simulink model "NetworkModelSimpleIntersectionSimpleDroneModel"  (R2018b)
settings: Solver=VariableStepAuto  StartTime=tStart  StopTime=tFinal  FixedStep=0.001  RelTol=1e-3
undefined symbols (not defined in the file or in its folder): bx, by, ConflictDrone1andDrone2, ConflictDrone1andDrone3, ConflictDrone1andDrone4, ConflictDrone2andDrone3, ConflictDrone2andDrone4, ConflictDrone3andDrone4, deltaVx1, deltaVx2, deltaVx3, deltaVx4, deltaVy1, deltaVy2, deltaVy3, deltaVy4, m, VelocityStarX1, VelocityStarX2, VelocityStarX3, VelocityStarX4, VelocityStarY1, VelocityStarY2, VelocityStarY3, VelocityStarY4, vx10, vx20, vx30, vx40, vy10, vy20, vy30, vy40, x10, x20, x30, x40, y10, y20, y30, y40
libraries: simulink x9
settings Model: Creator=CowUser  LastModifiedBy=CowUser

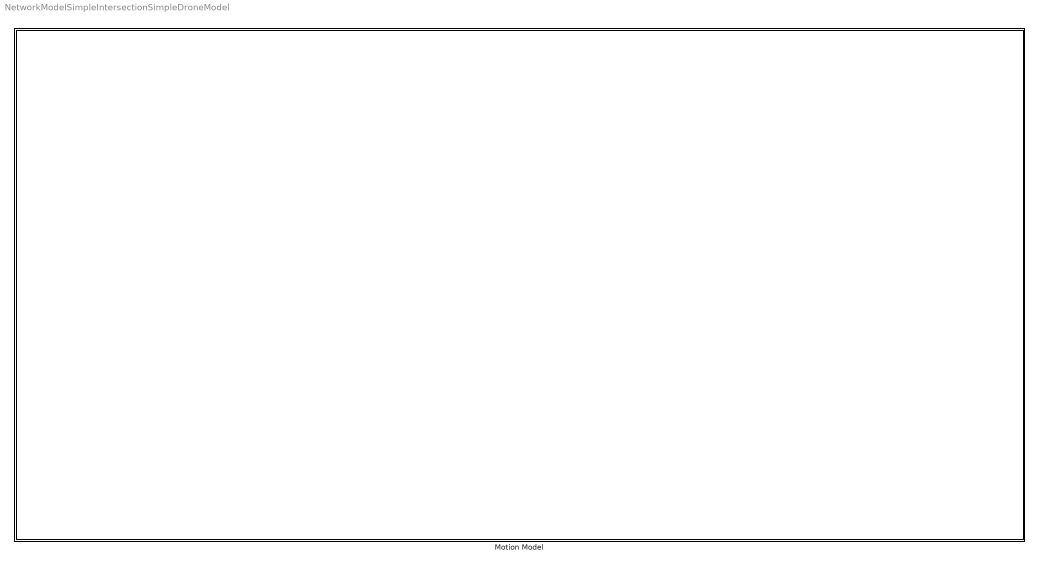
== system NetworkModelSimpleIntersectionSimpleDroneModel ==
  Motion Model : Subsystem

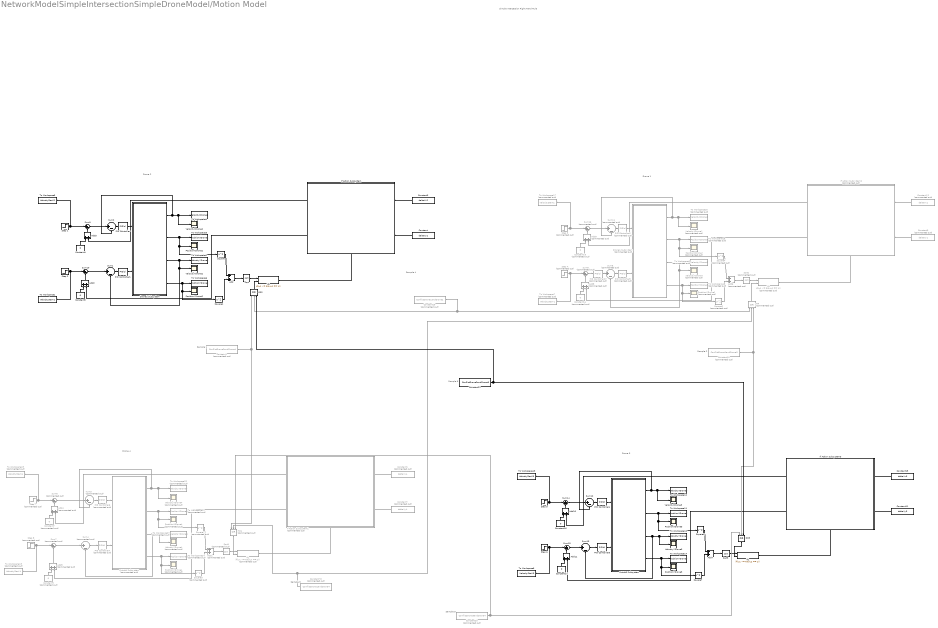
== system NetworkModelSimpleIntersectionSimpleDroneModel/Motion Model ==
  note: Drone 2
  note: Simple Intersection
      |
      | Right Hand Rule
  note: Drone 4
  note: Sample 1
  note: Drone 1
  note: Drone 3
  note: Sample 2
  note: Sample 3
  note: Sample 4
  note: Sample 5
  note: Sample 6
  Add{,2..3,7,10..11} (6 alike) : Sum
  Add{1,4..6,8..9} (6 alike) : Sum  Commented=on
  Constant : Constant  Value=deltaVy2
  Constant1 : Constant  Commented=on  Value=ConflictDrone2andDrone4
  Constant10 : Constant  Commented=on  Value=ConflictDrone1andDrone3
  Constant11 : Constant  Value=deltaVy3
  Constant12 : Constant  Commented=on  Value=deltaVx1
  Constant{7..8,13..14} (4 alike) : Constant  Commented=on  Value=0
  Constant15 : Constant  Value=deltaVx3
  Constant{4..5,16..17} (4 alike) : Constant  Value=0
  Constant18 : Constant  Commented=on  Value=ConflictDrone1andDrone4
  Constant19 : Constant  Commented=on  Value=ConflictDrone1andDrone2
  Constant2 : Constant  Commented=on  Value=deltaVy4
  Constant20 : Constant  Commented=on  Value=ConflictDrone3andDrone4
  Constant21 : Constant  Value=ConflictDrone2andDrone3
  Constant3 : Constant  Value=deltaVx2
  Constant6 : Constant  Commented=on  Value=deltaVx4
  Constant9 : Constant  Commented=on  Value=deltaVy1
  "Drone1 Subsystem " : Subsystem  Commented=on
  "Drone2 Subsystem " : Subsystem
  Drone3 Subsystem : Subsystem
  "Drone4 Subsystem " : Subsystem  Commented=on
  If Action Subsystem : Subsystem  TreatAsAtomicUnit=on
  If Action Subsystem1 : Subsystem  Commented=on  TreatAsAtomicUnit=on
  If Action Subsystem2 : Subsystem  Commented=on  TreatAsAtomicUnit=on
  If Action Subsystem3 : Subsystem  TreatAsAtomicUnit=on
  If1 : If  Commented=on  NumInputs=2  IfExpression=(u1 <= R)&(u2 == 1)  ShowElse=off
  If2 : If  NumInputs=2  IfExpression=(u1 <= R)&(u2 == 1)  ShowElse=off
  If3 : If  NumInputs=2  IfExpression=(u1 <= R)&(u2 == 1)  ShowElse=off
  If4 : If  Commented=on  NumInputs=2  IfExpression=(u1 <= R)&(u2 == 1)  ShowElse=off
  OR : Logic  Commented=on  Operator=OR  Inputs=3  IconShape=distinctive  AllPortsSameDT=off  OutDataTypeStr='double'
  OR1 : Logic  Commented=on  Operator=OR  Inputs=3  IconShape=distinctive  AllPortsSameDT=off  OutDataTypeStr='double'
  OR2 : Logic  Operator=OR  Inputs=3  IconShape=distinctive  AllPortsSameDT=off  OutDataTypeStr='double'
  OR3 : Logic  Operator=OR  Inputs=3  IconShape=distinctive  AllPortsSameDT=off  OutDataTypeStr='double'
  PID Controller{,1,4..5} (4 alike) : simulink/Continuous/PID Controller  Controller=PID  Form=Parallel  TimeDomain=Continuous-time  SampleTime=-1  IntegratorMethod=Forward Euler  FilterMethod=Forward Euler  ControllerParametersSource=internal  P=800  I=40  D=1  UseFilter=on  N=100  TunerSelectOption=Transfer Function Based (PID Tuner App)  InitialConditionSource=internal  InitialConditionForIntegrator=0  InitialConditionForFilter=0  DifferentiatorICPrevScaledInput=0  ExternalReset=none  TrackingMode=off  Kt=1  LimitOutput=off  UpperSaturationLimit=inf  LowerSaturationLimit=-inf  LinearizeAsGain=on  AntiWindupMode=none  Kb=1  POutMin=[]  POutMax=[]  IOutMin=[]  IOutMax=[]  DOutMin=[]  DOutMax=[]  NOutMin=[]  NOutMax=[]  SumOutMin=[]  SumOutMax=[]  SaturationOutMin=[]  SaturationOutMax=[]  PParamMin=[]  PParamMax=[]  IParamMin=[]  IParamMax=[]  DParamMin=[]  DParamMax=[]  NParamMin=[]  NParamMax=[]  KbParamMin=[]  KbParamMax=[]  KtParamMin=[]  KtParamMax=[]  KbOutMin=[]  KbOutMax=[]  KtOutMin=[]  KtOutMax=[]  IntegratorOutMin=[]  IntegratorOutMax=[]  FilterOutMin=[]  FilterOutMax=[]  SumI1OutMin=[]  SumI1OutMax=[]  SumI2OutMin=[]  SumI2OutMax=[]  SumI3OutMin=[]  SumI3OutMax=[]  SumI4OutMin=[]  SumI4OutMax=[]  SumDOutMin=[]  SumDOutMax=[]  DifferentiatorOutMin=[]  DifferentiatorOutMax=[]  FilterDiffOutCoefMin=[]  FilterDiffOutCoefMax=[]  ReciprocalOutMin=[]  ReciprocalOutMax=[]  SumDenOutMin=[]  SumDenOutMax=[]  SumNumOutMin=[]  SumNumOutMax=[]  DivideOutMin=[]  DivideOutMax=[]  IntegratorContinuousStateAttributes=''  IntegratorStateMustResolveToSignalObject=off  IntegratorRTWStateStorageClass=Auto  FilterContinuousStateAttributes=''  FilterStateMustResolveToSignalObject=off  FilterRTWStateStorageClass=Auto  ParallelPVariant=InternalParameters  IdealPVariant=Disabled  IVariant=InternalParameters  DVariant=InternalParameters  IntegratorVariant=Continuous  SatVariant=Disabled  AWVariant=Passthrough  PCopyVariant=Disabled  TRVariant=Disabled  FdbkBlocksVariant=Forward  IdealPFdbkVariant=Disabled  SatFdbkVariant=Disabled  DerivativeFilterVariant=ContFilter  NVariant=InternalParameters  NCopyVariant=Disabled  FilterICVariant=InternalICsFilter  IntegratorICVariant=InternalICs  ExternalResetVariant=Disabled  TRSumVariant=Passthrough  SumFdbkVariant=Disabled  SumVariant=Sum_PID
  PID Controller{2..3,6..7,10} (5 alike) : simulink/Continuous/PID Controller  Commented=on  Controller=PID  Form=Parallel  TimeDomain=Continuous-time  SampleTime=-1  IntegratorMethod=Forward Euler  FilterMethod=Forward Euler  ControllerParametersSource=internal  P=800  I=40  D=1  UseFilter=on  N=100  TunerSelectOption=Transfer Function Based (PID Tuner App)  InitialConditionSource=internal  InitialConditionForIntegrator=0  InitialConditionForFilter=0  DifferentiatorICPrevScaledInput=0  ExternalReset=none  TrackingMode=off  Kt=1  LimitOutput=off  UpperSaturationLimit=inf  LowerSaturationLimit=-inf  LinearizeAsGain=on  AntiWindupMode=none  Kb=1  POutMin=[]  POutMax=[]  IOutMin=[]  IOutMax=[]  DOutMin=[]  DOutMax=[]  NOutMin=[]  NOutMax=[]  SumOutMin=[]  SumOutMax=[]  SaturationOutMin=[]  SaturationOutMax=[]  PParamMin=[]  PParamMax=[]  IParamMin=[]  IParamMax=[]  DParamMin=[]  DParamMax=[]  NParamMin=[]  NParamMax=[]  KbParamMin=[]  KbParamMax=[]  KtParamMin=[]  KtParamMax=[]  KbOutMin=[]  KbOutMax=[]  KtOutMin=[]  KtOutMax=[]  IntegratorOutMin=[]  IntegratorOutMax=[]  FilterOutMin=[]  FilterOutMax=[]  SumI1OutMin=[]  SumI1OutMax=[]  SumI2OutMin=[]  SumI2OutMax=[]  SumI3OutMin=[]  SumI3OutMax=[]  SumI4OutMin=[]  SumI4OutMax=[]  SumDOutMin=[]  SumDOutMax=[]  DifferentiatorOutMin=[]  DifferentiatorOutMax=[]  FilterDiffOutCoefMin=[]  FilterDiffOutCoefMax=[]  ReciprocalOutMin=[]  ReciprocalOutMax=[]  SumDenOutMin=[]  SumDenOutMax=[]  SumNumOutMin=[]  SumNumOutMax=[]  DivideOutMin=[]  DivideOutMax=[]  IntegratorContinuousStateAttributes=''  IntegratorStateMustResolveToSignalObject=off  IntegratorRTWStateStorageClass=Auto  FilterContinuousStateAttributes=''  FilterStateMustResolveToSignalObject=off  FilterRTWStateStorageClass=Auto  ParallelPVariant=InternalParameters  IdealPVariant=Disabled  IVariant=InternalParameters  DVariant=InternalParameters  IntegratorVariant=Continuous  SatVariant=Disabled  AWVariant=Passthrough  PCopyVariant=Disabled  TRVariant=Disabled  FdbkBlocksVariant=Forward  IdealPFdbkVariant=Disabled  SatFdbkVariant=Disabled  DerivativeFilterVariant=ContFilter  NVariant=InternalParameters  NCopyVariant=Disabled  FilterICVariant=InternalICsFilter  IntegratorICVariant=InternalICs  ExternalResetVariant=Disabled  TRSumVariant=Passthrough  SumFdbkVariant=Disabled  SumVariant=Sum_PID
  PositionXDrone1 : Scope  Commented=on
  PositionXDrone2 : Scope
  PositionXDrone3 : Scope
  PositionXDrone4 : Scope  Commented=on
  PositionYDrone1 : Scope  Commented=on
  PositionYDrone2 : Scope
  PositionYDrone3 : Scope
  PositionYDrone4 : Scope  Commented=on
  Sqrt : Sqrt  SaturateOnIntegerOverflow=on
  Sqrt1 : Sqrt  Commented=on  SaturateOnIntegerOverflow=on
  Sqrt2 : Sqrt  Commented=on  SaturateOnIntegerOverflow=on
  Sqrt3 : Sqrt  SaturateOnIntegerOverflow=on
  Square{,1,6..7} (4 alike) : Math  Operator=square  SaturateOnIntegerOverflow=on
  Square{2..5} (4 alike) : Math  Commented=on  Operator=square  SaturateOnIntegerOverflow=on
  Step 1 : Step  Time=0  After=VelocityStarX2  SampleTime=0
  Step 2 : Step  Time=0  After=VelocityStarY2  SampleTime=0
  Step 3 : Step  Commented=on  Time=0  After=VelocityStarX1  SampleTime=0
  Step 4 : Step  Commented=on  Time=0  After=VelocityStarY1  SampleTime=0
  Step 5 : Step  Time=0  After=VelocityStarX3  SampleTime=0
  Step 6 : Step  Time=0  After=VelocityStarY3  SampleTime=0
  Step 7 : Step  Commented=on  Time=0  After=VelocityStarX4  SampleTime=0
  Step 8 : Step  Commented=on  Time=0  After=VelocityStarY4  SampleTime=0
  Sum{1..2,9..10,12..15} (8 alike) : Sum  Inputs=|+-
  Sum{3..8,11,16} (8 alike) : Sum  Commented=on  Inputs=|+-
  To Workspace1 : ToWorkspace  VariableName=VelocityStarY2  SampleTime=-1
  To Workspace10 : ToWorkspace  VariableName=VelocityYDrone3  SampleTime=-1
  To Workspace11 : ToWorkspace  VariableName=PositionXDrone3  SampleTime=-1
  To Workspace12 : ToWorkspace  VariableName=VelocityXDrone3  SampleTime=-1
  To Workspace13 : ToWorkspace  VariableName=VelocityStarX3  SampleTime=-1
  To Workspace14 : ToWorkspace  VariableName=PositionYDrone3  SampleTime=-1
  To Workspace15 : ToWorkspace  Commented=on  VariableName=PositionXDrone1  SampleTime=-1
  To Workspace16 : ToWorkspace  Commented=on  VariableName=VelocityXDrone1  SampleTime=-1
  To Workspace17 : ToWorkspace  Commented=on  VariableName=VelocityStarX1  SampleTime=-1
  To Workspace18 : ToWorkspace  Commented=on  VariableName=PositionYDrone1  SampleTime=-1
  To Workspace19 : ToWorkspace  Commented=on  VariableName=VelocityStarY4  SampleTime=-1
  To Workspace2 : ToWorkspace  VariableName=VelocityYDrone2  SampleTime=-1
  To Workspace20 : ToWorkspace  Commented=on  VariableName=VelocityYDrone4  SampleTime=-1
  To Workspace21 : ToWorkspace  Commented=on  VariableName=PositionXDrone4  SampleTime=-1
  To Workspace22 : ToWorkspace  Commented=on  VariableName=VelocityXDrone4  SampleTime=-1
  To Workspace23 : ToWorkspace  Commented=on  VariableName=VelocityStarX4  SampleTime=-1
  To Workspace24 : ToWorkspace  Commented=on  VariableName=PositionYDrone4  SampleTime=-1
  To Workspace3 : ToWorkspace  VariableName=PositionXDrone2  SampleTime=-1
  To Workspace4 : ToWorkspace  VariableName=VelocityXDrone2  SampleTime=-1
  To Workspace5 : ToWorkspace  VariableName=VelocityStarX2  SampleTime=-1
  To Workspace6 : ToWorkspace  VariableName=PositionYDrone2  SampleTime=-1
  To Workspace7 : ToWorkspace  Commented=on  VariableName=VelocityStarY1  SampleTime=-1
  To Workspace8 : ToWorkspace  VariableName=VelocityStarY3  SampleTime=-1
  To Workspace9 : ToWorkspace  Commented=on  VariableName=VelocityYDrone1  SampleTime=-1
  VelocityXDrone1 : Scope  Commented=on
  VelocityXDrone2 : Scope
  VelocityXDrone3 : Scope
  VelocityXDrone4 : Scope  Commented=on
  VelocityYDrone1 : Scope  Commented=on
  VelocityYDrone2 : Scope
  VelocityYDrone3 : Scope
  VelocityYDrone4 : Scope  Commented=on
  wires:
  "Drone2 Subsystem "/3(VelocityY) -> Sum1/2, VelocityYDrone2/1, To Workspace2/1
  Sum1/1 -> PID Controller1/1
  PID Controller/1 -> "Drone2 Subsystem "/1(InputForceX)
  "Drone2 Subsystem "/4(PositionY) -> Square1/1, PositionYDrone2/1, To Workspace6/1
  "Drone2 Subsystem "/2(PositionX) -> Square/1, PositionXDrone2/1, To Workspace3/1
  PID Controller1/1 -> "Drone2 Subsystem "/2(InputForceY)
  "Drone2 Subsystem "/1(VelocityX) -> VelocityXDrone2/1, To Workspace4/1, Sum2/2
  Step 7/1 -> Sum6/1, To Workspace23/1
  Step 8/1 -> To Workspace19/1, Sum7/1
  Square/1 -> Add/1
  Square1/1 -> Add/2
  Add/1 -> Sqrt/1
  Sqrt/1 -> If3/1
  Square2/1 -> Add1/1
  Add1/1 -> Sqrt1/1
  "Drone4 Subsystem "/2(PositionXTEST) -> Square2/1, PositionXDrone4/1, To Workspace21/1
  Square3/1 -> Add1/2
  "Drone4 Subsystem "/4(PositionYTEST) -> Square3/1, PositionYDrone4/1, To Workspace24/1
  Sqrt1/1 -> If1/1
  Sum2/1 -> PID Controller/1
  Constant/1 -> If Action Subsystem/2(deltaVy2)
  Constant3/1 -> If Action Subsystem/1(deltaVx2)
  Step 1/1 -> Sum9/1, To Workspace5/1
  Sum10/1 -> Sum1/1
  Step 2/1 -> Sum10/1, To Workspace1/1
  If Action Subsystem/1(dVx2) -> Add3/2
  If Action Subsystem/2(dVy2) -> Add2/2
  If3/1 -> If Action Subsystem/Action
  Constant4/1 -> Add3/1
  Constant5/1 -> Add2/1
  Add2/1 -> Sum10/2
  Constant1/1 -> OR1/1, OR2/1
  If1/1 -> If Action Subsystem1/Action
  If Action Subsystem1/1(dVx4) -> Add4/2
  Constant2/1 -> If Action Subsystem1/2(deltaVy4)
  Constant6/1 -> If Action Subsystem1/1(deltaVx4)
  Add4/1 -> Sum6/2
  Constant7/1 -> Add4/1
  Sum3/1 -> PID Controller6/1
  "Drone4 Subsystem "/1(VelocityXTEST) -> Sum3/2, To Workspace22/1, VelocityXDrone4/1
  Constant8/1 -> Add5/1
  If Action Subsystem1/2(dVy4) -> Add5/2
  "Drone4 Subsystem "/3(VelocityYTEST) -> Sum4/2, VelocityYDrone4/1, To Workspace20/1
  Sum4/1 -> PID Controller7/1
  Add3/1 -> Sum9/2
  Sum9/1 -> Sum2/1
  Step 3/1 -> Sum16/1, To Workspace17/1
  Add9/1 -> Sum16/2
  "Drone1 Subsystem "/4(PositionY) -> Square5/1, PositionYDrone1/1, To Workspace18/1
  Drone3 Subsystem/3(VelocityY) -> Sum13/2, VelocityYDrone3/1, To Workspace10/1
  Constant17/1 -> Add11/1
  Add10/1 -> Sum14/2
  Sum15/1 -> Sum13/1
  If Action Subsystem3/2(dVy3) -> Add11/2
  PID Controller2/1 -> "Drone1 Subsystem "/1(InputForceX)
  Add11/1 -> Sum15/2
  Sum11/1 -> PID Controller2/1
  Constant10/1 -> OR3/2, OR/3
  If Action Subsystem2/1(dVx1) -> Add9/2
  Constant11/1 -> If Action Subsystem3/2(deltaVy3)
  Constant13/1 -> Add9/1
  Sqrt3/1 -> If2/1
  Constant16/1 -> Add10/1
  PID Controller3/1 -> "Drone1 Subsystem "/2(InputForceY)
  Add8/1 -> Sum8/2
  Drone3 Subsystem/1(VelocityX) -> Sum12/2, To Workspace12/1, VelocityXDrone3/1
  Constant14/1 -> Add8/1
  If2/1 -> If Action Subsystem3/Action
  If Action Subsystem3/1(dVx3) -> Add10/2
  Drone3 Subsystem/4(PositionY) -> Square7/1, PositionYDrone3/1, To Workspace14/1
  Constant12/1 -> If Action Subsystem2/1(deltaVx1)
  Constant15/1 -> If Action Subsystem3/1(deltaVx3)
  Step 4/1 -> Sum8/1, To Workspace7/1
  "Drone1 Subsystem "/2(PositionX) -> Square4/1, PositionXDrone1/1, To Workspace15/1
  Add7/1 -> Sqrt3/1
  Square6/1 -> Add7/1
  Square5/1 -> Add6/2
  Constant9/1 -> If Action Subsystem2/2(deltaVy1)
  Square7/1 -> Add7/2
  Sum13/1 -> PID Controller5/1
  Drone3 Subsystem/2(PositionX) -> Square6/1, PositionXDrone3/1, To Workspace11/1
  Sum14/1 -> Sum12/1
  Step 5/1 -> Sum14/1, To Workspace13/1
  Sum12/1 -> PID Controller4/1
  Step 6/1 -> To Workspace8/1, Sum15/1
  Sum5/1 -> PID Controller3/1
  Sqrt2/1 -> If4/1
  PID Controller4/1 -> Drone3 Subsystem/1(InputForceX)
  Add6/1 -> Sqrt2/1
  PID Controller5/1 -> Drone3 Subsystem/2(InputForceY)
  "Drone1 Subsystem "/3(VelocityY) -> Sum5/2, VelocityYDrone1/1, To Workspace9/1
  If Action Subsystem2/2(dVy1) -> Add8/2
  Square4/1 -> Add6/1
  If4/1 -> If Action Subsystem2/Action
  "Drone1 Subsystem "/1(VelocityX) -> VelocityXDrone1/1, To Workspace16/1, Sum11/2
  OR/1 -> If4/2
  Constant18/1 -> OR/2, OR1/2
  OR1/1 -> If1/2
  OR2/1 -> If3/2
  Constant19/1 -> OR2/2, OR/1
  Constant20/1 -> OR3/1, OR1/3
  OR3/1 -> If2/2
  Constant21/1 -> OR3/3, OR2/3
  Sum6/1 -> Sum3/1
  PID Controller10/1 -> Sum5/1
  Sum8/1 -> PID Controller10/1
  Sum16/1 -> Sum11/1
  Add5/1 -> Sum7/2
  Sum7/1 -> Sum4/1
  PID Controller6/1 -> "Drone4 Subsystem "/1(InputForceXTEST)
  PID Controller7/1 -> "Drone4 Subsystem "/2(InputForceYTEST)

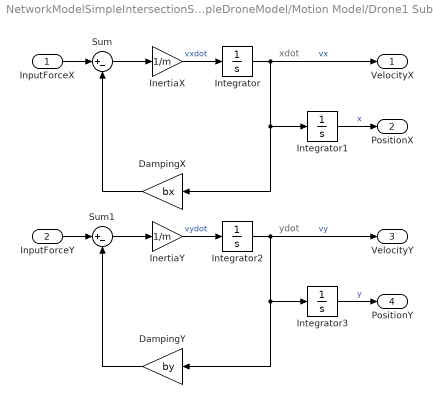
== system NetworkModelSimpleIntersectionSimpleDroneModel/Motion Model/Drone1 Subsystem  ==
  note: xdot
  note: ydot
  InputForceX : Inport
  InputForceY : Inport  Port=2
  "DampingX " : Gain  Gain=bx
  DampingY : Gain  Gain=by
  InertiaX : Gain  Gain=1/m
  InertiaY : Gain  Gain=1/m
  Integrator : Integrator  InitialCondition=vx10
  Integrator1 : Integrator  InitialCondition=x10
  Integrator2 : Integrator  InitialCondition=vy10
  Integrator3 : Integrator  InitialCondition=y10
  Sum : Sum  Inputs=|+-
  Sum1 : Sum  Inputs=|+-
  VelocityX : Outport
  PositionX : Outport  Port=2
  VelocityY : Outport  Port=3
  PositionY : Outport  Port=4
  wires:
  InputForceX/1 -> Sum/1
  InertiaX/1 -> Integrator/1  "vxdot"
  Sum/1 -> InertiaX/1
  Integrator/1 -> VelocityX/1, Integrator1/1, "DampingX "/1  "vx"
  "DampingX "/1 -> Sum/2
  Integrator1/1 -> PositionX/1  "x"
  DampingY/1 -> Sum1/2
  Sum1/1 -> InertiaY/1
  InertiaY/1 -> Integrator2/1  "vydot"
  Integrator3/1 -> PositionY/1  "y"
  InputForceY/1 -> Sum1/1
  Integrator2/1 -> VelocityY/1, Integrator3/1, DampingY/1  "vy"

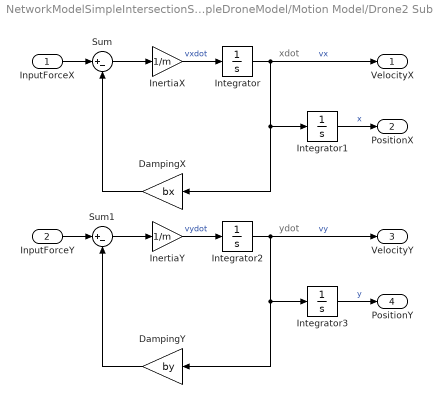
== system NetworkModelSimpleIntersectionSimpleDroneModel/Motion Model/Drone2 Subsystem  ==
  note: xdot
  note: ydot
  InputForceX : Inport
  InputForceY : Inport  Port=2
  "DampingX " : Gain  Gain=bx
  DampingY : Gain  Gain=by
  InertiaX : Gain  Gain=1/m
  InertiaY : Gain  Gain=1/m
  Integrator : Integrator  InitialCondition=vx20
  Integrator1 : Integrator  InitialCondition=x20
  Integrator2 : Integrator  InitialCondition=vy20
  Integrator3 : Integrator  InitialCondition=y20
  Sum : Sum  Inputs=|+-
  Sum1 : Sum  Inputs=|+-
  VelocityX : Outport
  PositionX : Outport  Port=2
  VelocityY : Outport  Port=3
  PositionY : Outport  Port=4
  wires:
  InputForceX/1 -> Sum/1
  InertiaX/1 -> Integrator/1  "vxdot"
  Sum/1 -> InertiaX/1
  Integrator/1 -> VelocityX/1, Integrator1/1, "DampingX "/1  "vx"
  "DampingX "/1 -> Sum/2
  Integrator1/1 -> PositionX/1  "x"
  DampingY/1 -> Sum1/2
  Sum1/1 -> InertiaY/1
  InertiaY/1 -> Integrator2/1  "vydot"
  Integrator3/1 -> PositionY/1  "y"
  InputForceY/1 -> Sum1/1
  Integrator2/1 -> VelocityY/1, Integrator3/1, DampingY/1  "vy"

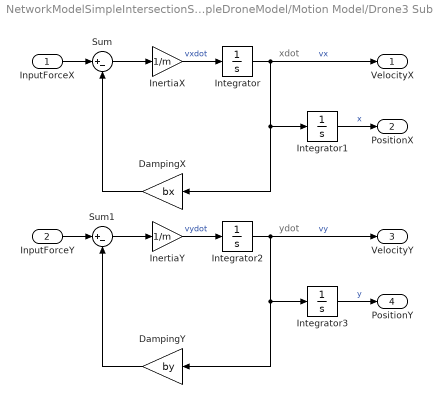
== system NetworkModelSimpleIntersectionSimpleDroneModel/Motion Model/Drone3 Subsystem ==
  note: xdot
  note: ydot
  InputForceX : Inport
  InputForceY : Inport  Port=2
  "DampingX " : Gain  Gain=bx
  DampingY : Gain  Gain=by
  InertiaX : Gain  Gain=1/m
  InertiaY : Gain  Gain=1/m
  Integrator : Integrator  InitialCondition=vx30
  Integrator1 : Integrator  InitialCondition=x30
  Integrator2 : Integrator  InitialCondition=vy30
  Integrator3 : Integrator  InitialCondition=y30
  Sum : Sum  Inputs=|+-
  Sum1 : Sum  Inputs=|+-
  VelocityX : Outport
  PositionX : Outport  Port=2
  VelocityY : Outport  Port=3
  PositionY : Outport  Port=4
  wires:
  InputForceX/1 -> Sum/1
  InertiaX/1 -> Integrator/1  "vxdot"
  Sum/1 -> InertiaX/1
  Integrator/1 -> VelocityX/1, Integrator1/1, "DampingX "/1  "vx"
  "DampingX "/1 -> Sum/2
  Integrator1/1 -> PositionX/1  "x"
  DampingY/1 -> Sum1/2
  Sum1/1 -> InertiaY/1
  InertiaY/1 -> Integrator2/1  "vydot"
  Integrator3/1 -> PositionY/1  "y"
  InputForceY/1 -> Sum1/1
  Integrator2/1 -> VelocityY/1, Integrator3/1, DampingY/1  "vy"

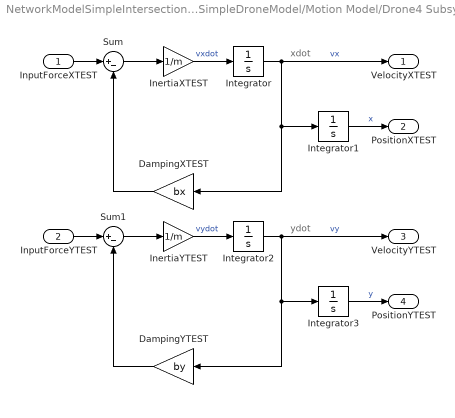
== system NetworkModelSimpleIntersectionSimpleDroneModel/Motion Model/Drone4 Subsystem  ==
  note: ydot
  note: xdot
  InputForceXTEST : Inport
  InputForceYTEST : Inport  Port=2
  "DampingXTEST " : Gain  Gain=bx
  DampingYTEST : Gain  Gain=by
  InertiaXTEST : Gain  Gain=1/m
  InertiaYTEST : Gain  Gain=1/m
  Integrator : Integrator  InitialCondition=vx40
  Integrator1 : Integrator  InitialCondition=x40
  Integrator2 : Integrator  InitialCondition=vy40
  Integrator3 : Integrator  InitialCondition=y40
  Sum : Sum  Inputs=|+-
  Sum1 : Sum  Inputs=|+-
  VelocityXTEST : Outport
  PositionXTEST : Outport  Port=2
  VelocityYTEST : Outport  Port=3
  PositionYTEST : Outport  Port=4
  wires:
  InputForceYTEST/1 -> Sum1/1
  Integrator3/1 -> PositionYTEST/1  "y"
  Integrator2/1 -> VelocityYTEST/1, Integrator3/1, DampingYTEST/1  "vy"
  Integrator/1 -> VelocityXTEST/1, Integrator1/1, "DampingXTEST "/1  "vx"
  Sum1/1 -> InertiaYTEST/1
  "DampingXTEST "/1 -> Sum/2
  InertiaXTEST/1 -> Integrator/1  "vxdot"
  InputForceXTEST/1 -> Sum/1
  Integrator1/1 -> PositionXTEST/1  "x"
  DampingYTEST/1 -> Sum1/2
  Sum/1 -> InertiaXTEST/1
  InertiaYTEST/1 -> Integrator2/1  "vydot"

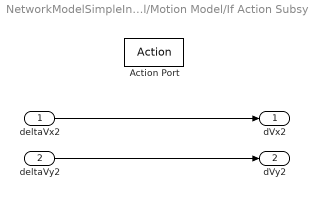
== system NetworkModelSimpleIntersectionSimpleDroneModel/Motion Model/If Action Subsystem ==
  deltaVx2 : Inport
  deltaVy2 : Inport  Port=2
  Action Port : ActionPort  ActionType=then
  dVx2 : Outport
  dVy2 : Outport  Port=2
  wires:
  deltaVx2/1 -> dVx2/1
  deltaVy2/1 -> dVy2/1

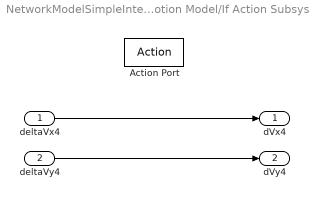
== system NetworkModelSimpleIntersectionSimpleDroneModel/Motion Model/If Action Subsystem1 ==
  deltaVx4 : Inport
  deltaVy4 : Inport  Port=2
  Action Port : ActionPort  ActionType=then
  dVx4 : Outport
  dVy4 : Outport  Port=2
  wires:
  deltaVx4/1 -> dVx4/1
  deltaVy4/1 -> dVy4/1

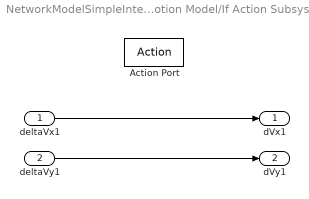
== system NetworkModelSimpleIntersectionSimpleDroneModel/Motion Model/If Action Subsystem2 ==
  deltaVx1 : Inport
  deltaVy1 : Inport  Port=2
  Action Port : ActionPort  ActionType=then
  dVx1 : Outport
  dVy1 : Outport  Port=2
  wires:
  deltaVx1/1 -> dVx1/1
  deltaVy1/1 -> dVy1/1

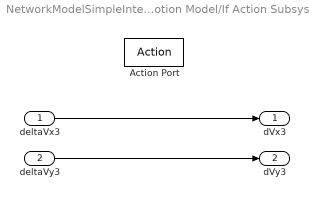
== system NetworkModelSimpleIntersectionSimpleDroneModel/Motion Model/If Action Subsystem3 ==
  deltaVx3 : Inport
  deltaVy3 : Inport  Port=2
  Action Port : ActionPort  ActionType=then
  dVx3 : Outport
  dVy3 : Outport  Port=2
  wires:
  deltaVx3/1 -> dVx3/1
  deltaVy3/1 -> dVy3/1
